simulink model "OriginalBatteryModel"  (R2024b)
settings: Solver=VariableStepAuto  StartTime=0.0  StopTime=3000  FixedStep=0.1  MaxStep=1  RelTol=1e-3
InitFcn:
  | load DOE_Data.mat;
model workspace (MAT data in the model file):
  SOCs1 = 0.5
undefined symbols (not defined in the file): AH, CurrLb_LUT, CurrUb_LUT, Np, s, SOCs, T_bkpts, Ts
libraries: fl_lib x6, nesl_utility x2, batt_lib x1, moduleExample_lib x1, simulink x1, SimscapeFluids_lib x1
settings Model: Creator=xiangchz  LastModifiedBy=msatra
settings OptimizationCC: ReuseModelBlockBuffer=off
settings RTWCC: GPUComputeCapability=3.5

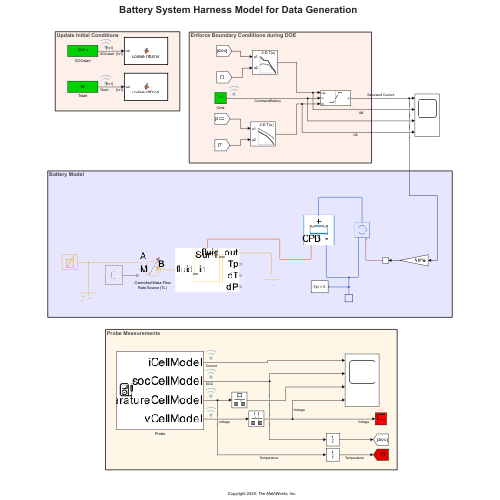
[thumbnail: Simulink's stored preview of the top-level diagram]
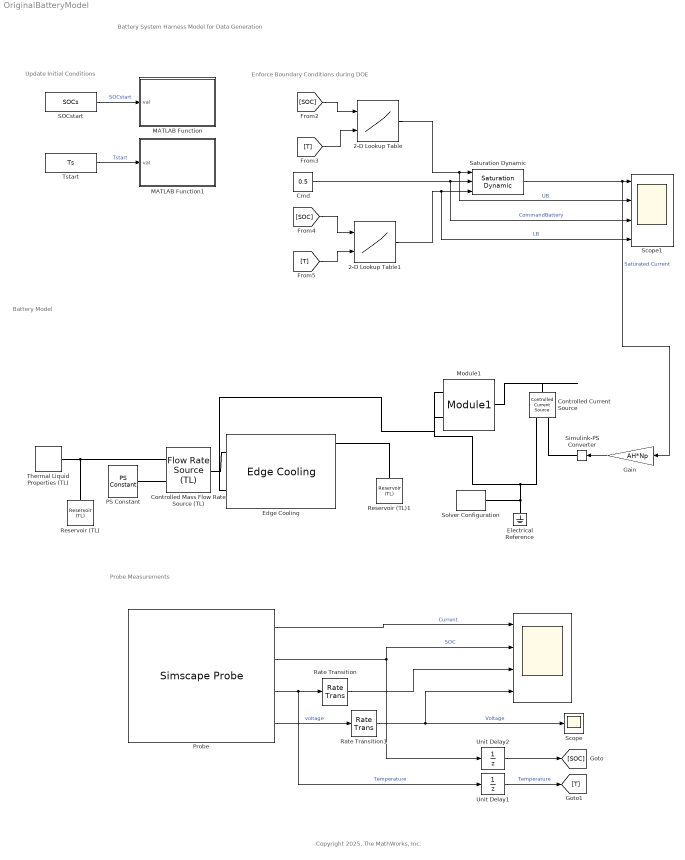
== system OriginalBatteryModel ==
  note: Copyright 2025, The MathWorks, Inc.
  note: Battery Model
  note: Update Initial Conditions
  note: Probe Measurements
  note: Battery System Harness Model for Data Generation
  note: Enforce Boundary Conditions during DOE
  " " : Scope  NumInputPorts=4
  2-D Lookup Table : Lookup_n-D  BreakpointsForDimension1=SOC_bkpts'  BreakpointsForDimension2=T_bkpts  Table=CurrUb_LUT  InternalRulePriority=Speed  RndMeth=Simplest
      settings: InputPortMap=u0,u1
  2-D Lookup Table1 : Lookup_n-D  BreakpointsForDimension1=SOC_bkpts'  BreakpointsForDimension2=T_bkpts  Table=CurrLb_LUT  InternalRulePriority=Speed  RndMeth=Simplest
      settings: InputPortMap=u0,u1
  Cmd : Constant  Value=0.5  SampleTime=0.1
  Controlled Current Source : fl_lib/Electrical/Electrical Sources/Controlled Current Source
  Controlled Mass Flow Rate Source (TL) : fl_lib/Thermal Liquid/Sources/Flow Rate Source (TL)  source_type=foundation.enum.constant_controlled.controlled  flow_type=foundation.enum.mass_volumetric_flow.mass  mass_flow=0 kg/s  volumetric_flow=0 m^3/s  power_spec=foundation.enum.power_spec.isentropic  area=0.01 m^2
  Edge Cooling : batt_lib/Thermal/Edge Cooling  plateConnectivity=simscape.battery.enum.thermal.coolingPlateConnectivity.singleSided  numBattThermalNodes1=module.ThermalNodes.Bottom.NumNodes  dimensionThermalNodes1=module.ThermalNodes.Bottom.Dimensions  locationThermalNodes1=module.ThermalNodes.Bottom.Locations  numBattThermalNodes2=1  dimensionThermalNodes2=ones(1, 2)  locationThermalNodes2=ones(1, 2)  plateDimX=2  plateDimY=5  plateTh=2e-3 m  plateThCond=20 W/(K*m)  plateDen=2500 kg/m^3  plateCp=447 J/(K*kg)  plateTemp_ini=278 K  Re_lam=2000  Re_tur=4000  Nu_lam=3.66  length_add=1e-3 m  shape_factor=64  selectEdgeOrientation=simscape.battery.enum.thermal.coolingEdgeDirection.alongY0  channelDia=5e-3 m  channelArea=2e-5 m^2  roughnessPipe=1.5e-05 m
      settings: InternalSimscapePortConfiguration="{\"Bottom\":[],\"Left\":[{\"id\":\"fluid_in\",\"label\":\"fluid_in\",\"type\":\"foundation.thermal_liquid.thermal_liquid\"}],\"Right\":[{\"id\":\"fluid_out\",\"label\":\"fluid_out\",\"type\":\"foundation.thermal_liquid.thermal_liquid\"},{\"id\":\"plotPlateT\",\"label\":\"Tp\",\"type\":\"output\"},{\"id\":\"tempSensor\",\"label\":\"dT\",\"type\":\"output\"},{\"id\":\"presSensor\",\"label\":\"dP\",\"type\":\"output\"}],\"Top\":[{\"id\":\"Side1\",\"label\":\"Surf1\",\"type\":\"foundation.thermal.thermal\"}]}"
  Electrical Reference : fl_lib/Electrical/Electrical Elements/Electrical Reference
  Gain : Gain  Gain=AH*Np
  MATLAB Function : MATLAB Function  TreatAsAtomicUnit=on
  MATLAB Function1 : MATLAB Function  TreatAsAtomicUnit=on
  Module1 : moduleExample_lib/Module1  SOC_vec=[0, .1, .25, .5, .75, .9, 1]  T_vec=[278, 293, 313] K  V0_mat=[3.49, 3.5, 3.51; 3.55, 3.57, 3.56; 3.62, 3.63, 3.64; 3.71, 3.71, 3.72; 3.91, 3.93, 3.94; 4.07, 4.08, 4.08; 4.19, 4.19, 4.19] V  V_range=[0, inf] V  R0_mat=[.0117, .0085, .009; .011, .0085, .009; .0114, .0087, .0092; .0107, .0082, .0088; .0107, .0083, .0091; .0113, .0085, .0089; .0116, .0085, .0089] Ohm  AH=27 A*hr  extrapolation_option=simscape.enum.extrapolation.nearest  R1_mat=[.0109, .0029, .0013; .0069, .0024, .0012; .0047, .0026, .0013; .0034, .0016, .001; .0033, .0023, .0014; .0033, .0018, .0011; .0028, .0017, .0011] Ohm  tau1_mat=[20, 36, 39; 31, 45, 39; 109, 105, 61; 36, 29, 26; 59, 77, 67; 40, 33, 29; 25, 39, 33] s  thermal_mass=100 J/K  CoolantResistance=1.2 K/W  P=4  S=10  iCellModel_specify=off  iCellModel_priority=None  iCellModel=0 A  iCellModel_nominal_specify=off  iCellModel_nominal_unit=A  iCellModel_nominal_value=1  vCellModel_specify=off  vCellModel_priority=None  vCellModel=0 V  vCellModel_nominal_specify=off  vCellModel_nominal_unit=V  vCellModel_nominal_value=1  socCellModel_specify=on  socCellModel_priority=High  socCellModel=SOCs  socCellModel_nominal_specify=off  socCellModel_nominal_unit=1  socCellModel_nominal_value=1  numCyclesCellModel_specify=off  numCyclesCellModel_priority=High  numCyclesCellModel=0  numCyclesCellModel_nominal_specify=off  numCyclesCellModel_nominal_unit=1  numCyclesCellModel_nominal_value=1  temperatureCellModel_specify=on  temperatureCellModel_priority=High  temperatureCellModel=Ts K  temperatureCellModel_nominal_specify=off  temperatureCellModel_nominal_unit=K  temperatureCellModel_nominal_value=1  vParallelAssembly_specify=off  vParallelAssembly_priority=None  vParallelAssembly=repmat(0, 10, 1) V  vParallelAssembly_nominal_specify=off  vParallelAssembly_nominal_unit=V  vParallelAssembly_nominal_value=1  socParallelAssembly_specify=off  socParallelAssembly_priority=None  socParallelAssembly=repmat(1, 10, 1)  socParallelAssembly_nominal_specify=off  socParallelAssembly_nominal_unit=1  socParallelAssembly_nominal_value=1
      settings: InternalSimscapePortConfiguration="{\"Bottom\":[{\"id\":\"n\",\"label\":\"-\",\"type\":\"foundation.electrical.electrical\"},{\"id\":\"BottomExtClnt\",\"label\":\"CPB\",\"type\":\"foundation.thermal.thermal\"}],\"Left\":[],\"Right\":[],\"Top\":[{\"id\":\"p\",\"label\":\"+\",\"type\":\"foundation.electrical.electrical\"}]}"
  PS Constant : fl_lib/Physical Signals/Sources/PS Constant  constant=0.2 kg/s
  Probe : SimscapeProbe  BoundBlock=440  Variables={iCellModel, socCellModel, temperatureCellModel, vCellModel}
  Rate Transition : RateTransition  InitialCondition=SOCs  OutPortSampleTime=0.1
  Rate Transition1 : RateTransition  InitialCondition=Ts  OutPortSampleTime=0.1
  Reservoir (TL) : fl_lib/Thermal Liquid/Elements/Reservoir (TL)  pressure_spec=foundation.enum.pressure_spec.atmospheric  reservoir_pressure=0.101325 MPa  reservoir_temperature=278 K  area=0.01 m^2
  Reservoir (TL)1 : fl_lib/Thermal Liquid/Elements/Reservoir (TL)  pressure_spec=foundation.enum.pressure_spec.atmospheric  reservoir_pressure=0.101325 MPa  reservoir_temperature=278 K  area=0.01 m^2
  SOCstart : Constant  Value=SOCs  VectorParams1D=off  SampleTime=0.1
  Saturation Dynamic : simulink/Discontinuities/Saturation Dynamic  OutMin=[]  OutMax=[]  OutDataTypeStr=Inherit: Same as second input  OutDataType=fixdt(1, 16)  OutScaling=2^-10  DoSatur=off
  Scope : Scope
  Scope1 : Scope  NumInputPorts=4
  Simulink-PS Converter : nesl_utility/Simulink-PS Converter  PhysicalDomain=network_engine_domain  SubClassName=ps_input  LeftPortType=input  RightPortType=output  PseudoPeriodic=off  Frequencies=[]  NoiseDistribution=none  NoiseParameters=[]  Unit=1  AffineConversion=off  FilteringAndDerivatives=provide  SimscapeFilterOrder=1  InputFilterTimeConstant=0.001  UdotUserProvided=0
  Solver Configuration : nesl_utility/Solver Configuration  PhysicalDomain=network_engine_domain  SubClassName=solver  LeftPortType=input  RightPortType=generic  Tones=[]  Harmonics=[]  SimulateNoise=off  Profile=off  UseLocalSampling=off  EnableSwitchedLinearOptims=on  FrequencyDomain=off  UseCCode=off  RelTol=0.001  AbsTol=0.001  MinStep=1e-09  ToWorkspace=off  RevertToSquareIcSolve=off  NumHomotopyIterations=100  PhasorMode=off  PhasorModeNumHarmonics=1  ConsistencySolver=NEWTON_XTOL_AFTER_FTOL  IndexReductionMethod=DerivativeReplacement  DoDC=off  ResidualTolerance=1e-09  ConsistencyTolSource=GLOBAL  ConsistencyAbsTol=0.001  ConsistencyRelTol=0.001  ConsistencyTolFactor=0.001  UseLocalSolver=off  LocalSolverChoice=NE_BACKWARD_EULER_ADVANCER  ResolveIndetEquations=on  FunctionEvalNumThread=1  LocalSolverSampleTime=0.001  DoFixedCost=off  MaxNonlinIter=3  MaxModeIter=2  ComputeImpulses=off  ImpulseIterations=2  LinearAlgebra=auto  LinearAlgebraNumThread=0  EquationFormulation=NE_TIME_EF  DelaysMemoryBudget=1024  AutomaticFiltering=on  FilteringTimeConstant=0.001  PartitionStorageMethod=AS_NEEDED  PartitionMemoryBudget=1024  PartitionMethod=ROBUST  MultibodyUseLocalSolver=off  MultibodyLocalSolverChoice=ODE1  MultibodyLocalSolverSampleTime=0.001
  Thermal Liquid Properties (TL) : SimscapeFluids_lib/Thermal Liquid/Utilities/Thermal Liquid Properties (TL)  fluid_list=fluids.thermal_liquid.utilities.enum.thermal_liquid_fluid_list.water  concentration_param_EG=fluids.thermal_liquid.utilities.enum.thermal_liquid_concentration.volume_fraction  concentration_param_PG=fluids.thermal_liquid.utilities.enum.thermal_liquid_concentration.volume_fraction  c_mass_SW=3.5e-3  c_mass_EG=0.1  c_mass_PG=0.1  c_mass_GL=0.1  c_vol_EG=0.1  c_vol_PG=0.1  beta_const_EG=2.1791 GPa  beta_const_PG=2.1791 GPa  beta_const_GL=2.1791 GPa  p_min_EG=0.01 MPa  p_min_PG=0.01 MPa  p_min_GL=0.01 MPa  p_max_EG=50 MPa  p_max_PG=50 MPa  p_max_GL=50 MPa  p_atm=0.101325 MPa  properties_range_check=simscape.enum.assert.action.error
  Tstart : Constant  Value=Ts  VectorParams1D=off  SampleTime=0.1
  Unit Delay1 : UnitDelay  InitialCondition=s(1,3)  SampleTime=-1  HasFrameUpgradeWarning=on
  Unit Delay2 : UnitDelay  InitialCondition=s(1,2)  SampleTime=-1  HasFrameUpgradeWarning=on
  wires:
  Probe/1 -> " "/1  "Current"
  Probe/3 -> Rate Transition/1, Unit Delay1/1  "Temperature"
  Gain/1 -> Simulink-PS Converter/1
  Probe/4 -> Rate Transition1/1  "voltage"
  Cmd/1 -> Scope1/3, Saturation Dynamic/2  "CommandBattery"
  Probe/2 -> Unit Delay2/1, " "/2  "SOC"
  [SOC] -> 2-D Lookup Table/1
  [T] -> 2-D Lookup Table/2
  2-D Lookup Table/1 -> Scope1/2, Saturation Dynamic/1  "UB"
  [SOC] -> 2-D Lookup Table1/1
  [T] -> 2-D Lookup Table1/2
  2-D Lookup Table1/1 -> Scope1/4, Saturation Dynamic/3  "LB"
  Saturation Dynamic/1 -> Gain/1, Scope1/1  "Saturated Current"
  Unit Delay2/1 -> [SOC]
  Rate Transition1/1 -> Scope/1, " "/4  "Voltage"
  Tstart/1 -> MATLAB Function1/1(val)  "Tstart"
  SOCstart/1 -> MATLAB Function/1(val)  "SOCstart"
  Rate Transition/1 -> " "/3
  Unit Delay1/1 -> [T]  "Temperature"
  connections:
  Controlled Current Source/RConn2 -- Module1/RConn1 -- Electrical Reference/LConn1 -- Solver Configuration/RConn1
  Controlled Mass Flow Rate Source (TL)/RConn1 -- Edge Cooling/LConn1
  Reservoir (TL)/LConn1 -- Thermal Liquid Properties (TL)/RConn1 -- Controlled Mass Flow Rate Source (TL)/LConn1
  PS Constant/RConn1 -- Controlled Mass Flow Rate Source (TL)/LConn2
  Edge Cooling/RConn1 -- Reservoir (TL)1/LConn1
  Module1/RConn2 -- Edge Cooling/LConn2
  Simulink-PS Converter/RConn1 -- Controlled Current Source/RConn1
  Module1/LConn1 -- Controlled Current Source/LConn1

== matlab function OriginalBatteryModel/MATLAB Function ==
  data: val input
function updateInitCond(val)
assignin('base', 'SOCs', val);

== matlab function OriginalBatteryModel/MATLAB Function1 ==
  data: val input
function updateInitCond(val)
assignin('base', 'Ts', val);
